simulink model "sim2"  (R2023a)
settings: Solver=ode8  StartTime=0.0  StopTime=50.0  FixedStep=0.001  RelTol=1e-3
values from neighbouring files (symbols this model uses):
  A = [ 0 1; -0.25 0]    [sim_data2.m]
  B = [0; 0]    [sim_data2.m]
  C = [1 0]    [sim_data2.m]
  D = [0]    [sim_data2.m]
  dt1 = 1/fs1    (= 0.2)    [sim_data1.m]    (also in sim_data2.m)
  system_disc1 = c2d(system_contin, dt1)    [sim_data2.m]
settings Model: Creator=ozar  LastModifiedBy=ozar

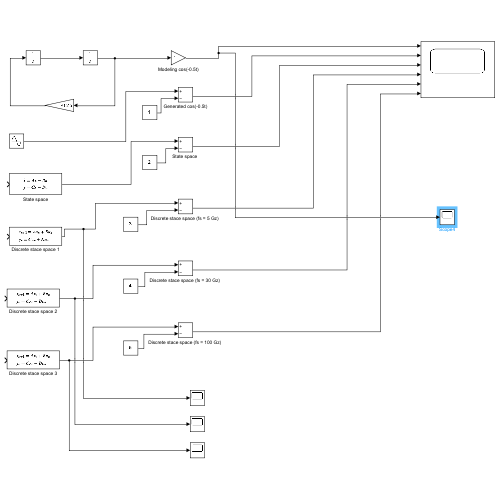
[thumbnail: Simulink's stored preview of the top-level diagram]
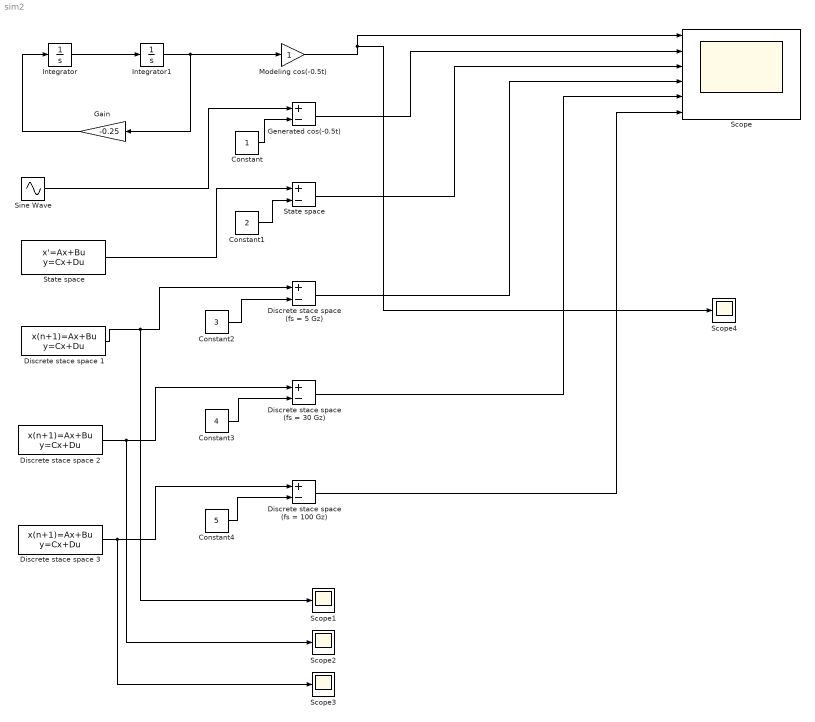
== system sim2 ==
  Constant : Constant
  Constant1 : Constant  Value=2
  Constant2 : Constant  Value=3
  Constant3 : Constant  Value=4
  Constant4 : Constant  Value=5
  "Discrete stace space (fs = 100 Gz) " : Sum  Inputs=+-
  "Discrete stace space (fs = 30 Gz) " : Sum  Inputs=+-
  "Discrete stace space (fs = 5 Gz) " : Sum  Inputs=+-
  Discrete stace space 1 : DiscreteStateSpace  A=system_disc1.A  B=system_disc1.B  C=system_disc1.C  D=system_disc1.D  InitialCondition=[1; 0]  SampleTime=dt1
  Discrete stace space 2 : DiscreteStateSpace  A=system_disc1.A  B=system_disc1.B  C=system_disc1.C  D=system_disc1.D  InitialCondition=[1; 0]  SampleTime=dt1
  Discrete stace space 3 : DiscreteStateSpace  A=system_disc1.A  B=system_disc1.B  C=system_disc1.C  D=system_disc1.D  InitialCondition=[1; 0]  SampleTime=dt1
  Gain : Gain  Gain=-0.25
  Generated cos(-0.5t) : Sum  Inputs=+-
  Integrator : Integrator
  Integrator1 : Integrator  InitialCondition=1
  Modeling cos(-0.5t) : Gain
  Scope : Scope  NumInputPorts=6
  Scope{1..4} (4 alike) : Scope
  Sine Wave : Sin  Frequency=0.5  Phase=pi/2  SampleTime=0
  State space : StateSpace  A=A  B=B  C=C  D=D  InitialCondition=[1; 0]
  "State space " : Sum  Inputs=+-
  wires:
  Integrator/1 -> Integrator1/1
  Gain/1 -> Integrator/1
  Integrator1/1 -> Gain/1, Modeling cos(-0.5t)/1
  Constant/1 -> Generated cos(-0.5t)/2
  Sine Wave/1 -> Generated cos(-0.5t)/1
  Generated cos(-0.5t)/1 -> Scope/2
  Modeling cos(-0.5t)/1 -> Scope4/1, Scope/1
  "State space "/1 -> Scope/3
  State space/1 -> "State space "/1
  Constant1/1 -> "State space "/2
  Constant2/1 -> "Discrete stace space (fs = 5 Gz) "/2
  "Discrete stace space (fs = 5 Gz) "/1 -> Scope/4
  Discrete stace space 2/1 -> Scope2/1, "Discrete stace space (fs = 30 Gz) "/1
  "Discrete stace space (fs = 30 Gz) "/1 -> Scope/5
  Constant3/1 -> "Discrete stace space (fs = 30 Gz) "/2
  Constant4/1 -> "Discrete stace space (fs = 100 Gz) "/2
  "Discrete stace space (fs = 100 Gz) "/1 -> Scope/6
  Discrete stace space 3/1 -> Scope3/1, "Discrete stace space (fs = 100 Gz) "/1
  Discrete stace space 1/1 -> Scope1/1, "Discrete stace space (fs = 5 Gz) "/1
